simulink model "para_amanha"  (R2013a)
settings: Solver=ode45  StartTime=0.0  StopTime=10.0  RelTol=1e-3
libraries: aerolibtransform2 x3
settings Model: Creator=Daniel  LastModifiedBy=Administrator

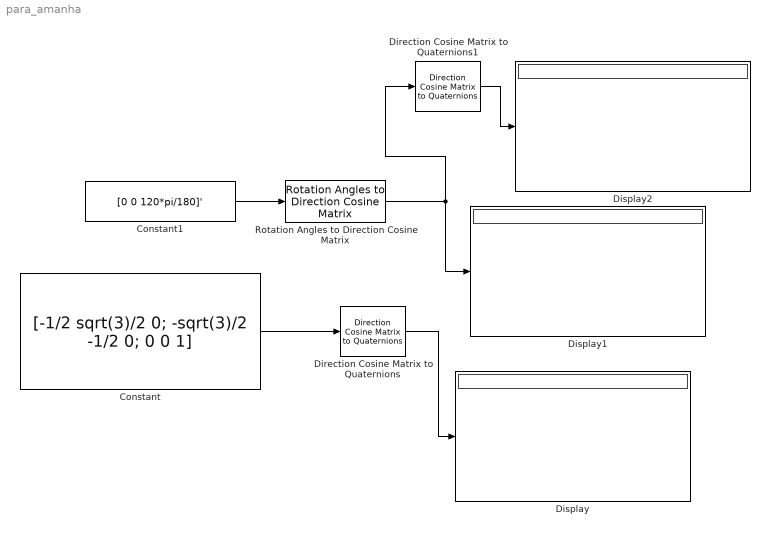
== system para_amanha ==
  Constant : Constant  Value="[-1/2 sqrt(3)/2  0; -sqrt(3)/2 -1/2 0; 0 0 1]"
  Constant1 : Constant  Value=[0 0 120*pi/180]'
  Direction Cosine Matrix to Quaternions : aerolibtransform2/Direction Cosine Matrix  to Quaternions
  Direction Cosine Matrix to Quaternions1 : aerolibtransform2/Direction Cosine Matrix  to Quaternions
  Display : Display
  Display1 : Display
  Display2 : Display
  Rotation Angles to Direction Cosine Matrix : aerolibtransform2/Rotation Angles to Direction Cosine Matrix  rotationOrder=XYZ
  wires:
  Constant/1 -> Direction Cosine Matrix to Quaternions/1
  Direction Cosine Matrix to Quaternions/1 -> Display/1
  Rotation Angles to Direction Cosine Matrix/1 -> Direction Cosine Matrix to Quaternions1/1, Display1/1
  Constant1/1 -> Rotation Angles to Direction Cosine Matrix/1
  Direction Cosine Matrix to Quaternions1/1 -> Display2/1
